simulink model "Hinf_sym"  (R2023a)
settings: Solver=VariableStepAuto  StartTime=0.0  StopTime=100  RelTol=1e-3
InitFcn:
  | %Hinf_init
values from neighbouring files (symbols this model uses):
  C = [1 0 0 0; 0 1 0 0]    [Hinf_1DOF.m]    (also in Hinf_2DOFinit.m; Hinf_U_init.m; Hinf_WU_init.m; Hinf_init.m)
  dtheta_0 = 0    [Hinf_1DOF.m]    (also in Hinf_2DOFinit.m; Hinf_U_init.m; Hinf_WU_init.m; Hinf_init.m)
  dz_0 = 0    [Hinf_1DOF.m]    (also in Hinf_2DOFinit.m; Hinf_U_init.m; Hinf_WU_init.m; Hinf_init.m)
  fa_w = 0    [Hinf_1DOF.m]    (also in Hinf_2DOFinit.m; Hinf_U_init.m; Hinf_WU_init.m; Hinf_init.m)
  fm_w = s_param.g*s_param.m    [Hinf_1DOF.m]    (also in Hinf_2DOFinit.m; Hinf_U_init.m; Hinf_WU_init.m; Hinf_init.m)
  K = tf(ss(K.A,K.B,K.C,K.D))    [Hinf_U_init.m]    (also in Hinf_WU_init.m; Hinf_init.m = tf(K))
  Km1 = 1.1    [Hinf_1DOF.m]    (also in Hinf_2DOFinit.m; Hinf_U_init.m; Hinf_WU_init.m; Hinf_init.m)
  Km1_real = Km1 + std_dev_Km*randn(1,1)    [Hinf_1DOF.m]    (also in Hinf_2DOFinit.m; Hinf_U_init.m; Hinf_WU_init.m; Hinf_init.m)
  Km2 = 1.1    [Hinf_1DOF.m]    (also in Hinf_2DOFinit.m; Hinf_U_init.m; Hinf_WU_init.m; Hinf_init.m)
  Km2_real = Km2 + std_dev_Km*randn(1,1)    [Hinf_1DOF.m]    (also in Hinf_2DOFinit.m; Hinf_U_init.m; Hinf_WU_init.m; Hinf_init.m)
  omega_d1 = 1    [Hinf_init.m]
  omega_d2 = 1    [Hinf_init.m]
  omega_y1 = 1e3    (= 1000)    [Hinf_WU_init.m]    (also in Hinf_init.m)
  omega_y2 = 1e3    (= 1000)    [Hinf_WU_init.m]    (also in Hinf_init.m)
  T1 = 0.05    [Hinf_1DOF.m]    (also in Hinf_2DOFinit.m; Hinf_U_init.m; Hinf_WU_init.m; Hinf_init.m)
  T1_real = T1 + std_dev_T*randn(1,1)    [Hinf_1DOF.m]    (also in Hinf_2DOFinit.m; Hinf_U_init.m; Hinf_WU_init.m; Hinf_init.m)
  T2 = 0.15    [Hinf_1DOF.m]    (also in Hinf_2DOFinit.m; Hinf_U_init.m; Hinf_WU_init.m; Hinf_init.m)
  T2_real = T2 + std_dev_T*randn(1,1)    [Hinf_1DOF.m]    (also in Hinf_2DOFinit.m; Hinf_U_init.m; Hinf_WU_init.m; Hinf_init.m)
  theta_0_real = theta_0 + std_dev.theta_0*randn(1,1)    [Hinf_1DOF.m]    (also in Hinf_2DOFinit.m = theta_0+std_dev.theta_0*randn(1,1); Hinf_U_init.m = theta_0+std_dev.theta_0*randn(1,1); Hinf_WU_init.m = theta_0+std_dev.theta_0*randn(1,1); Hinf_init.m = theta_0+std_dev.theta_0*randn(1,1))
  theta_w = 0    [Hinf_1DOF.m]    (also in Hinf_2DOFinit.m; Hinf_U_init.m; Hinf_WU_init.m; Hinf_init.m)
  Tm1 = 1    [Hinf_1DOF.m]    (also in Hinf_2DOFinit.m; Hinf_U_init.m; Hinf_WU_init.m; Hinf_init.m)
  Tm1_real = Tm1 + std_dev_Tm*randn(1,1)    [Hinf_1DOF.m]    (also in Hinf_2DOFinit.m; Hinf_U_init.m; Hinf_WU_init.m; Hinf_init.m)
  Tm2 = 1    [Hinf_1DOF.m]    (also in Hinf_2DOFinit.m; Hinf_U_init.m; Hinf_WU_init.m; Hinf_init.m)
  Tm2_real = Tm2 + std_dev_Tm*randn(1,1)    [Hinf_1DOF.m]    (also in Hinf_2DOFinit.m; Hinf_U_init.m; Hinf_WU_init.m; Hinf_init.m)
  z_0_real = z_0 + std_dev.z_0*randn(1,1)    [Hinf_1DOF.m]    (also in Hinf_2DOFinit.m = z_0+std_dev.z_0*randn(1,1); Hinf_U_init.m = z_0+std_dev.z_0*randn(1,1); Hinf_WU_init.m = z_0+std_dev.z_0*randn(1,1); Hinf_init.m = z_0+std_dev.z_0*randn(1,1))
  z_w = 200    [Hinf_1DOF.m]    (also in Hinf_2DOFinit.m = 400; Hinf_U_init.m = 400; Hinf_WU_init.m = 400; Hinf_init.m = 400)
undefined symbols (not defined in the file or in its folder): s_param, s_param_r, std_dev
libraries: simulink x4
settings Model: Creator=franc  LastModifiedBy=franc

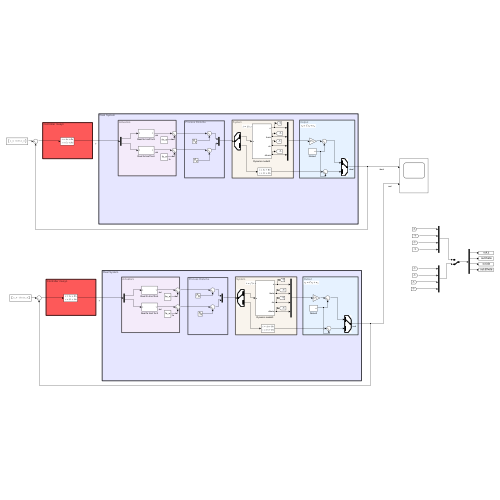
[thumbnail: Simulink's stored preview of the top-level diagram]
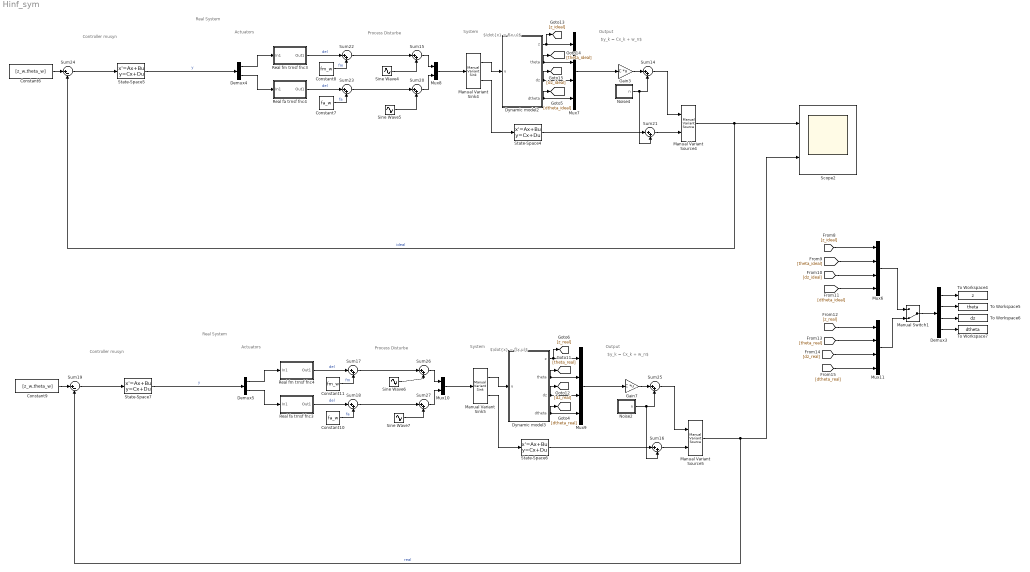
== system Hinf_sym ==
  note: $\dot{x} = f(x,u)$
  note: Controller musyn
  note: Real System
  note: Actuators
  note: Output
  note: Process Disturbe
  note: Controller musyn
  note: $y_k = Cx_k + w_n$
  note: System
  note: Process Disturbe
  note: $\dot{x} = f(x,u)$
  note: Actuators
  note: $y_k = Cx_k + w_n$
  note: Output
  note: System
  note: Real System
  Constant10 : Constant  Value=fa_w
  Constant11 : Constant  Value=fm_w
  Constant6 : Constant  Value=[z_w,theta_w]
  Constant7 : Constant  Value=fa_w
  Constant8 : Constant  Value=fm_w
  Constant9 : Constant  Value=[z_w,theta_w]
  Demux3 : Demux
  Demux4 : Demux  Outputs=2
  Demux5 : Demux  Outputs=2
  Dynamic model2 : Subsystem
  Dynamic model3 : Subsystem
  Gain3 : Gain  Gain=C  Multiplication=Matrix(K*u)
  Gain7 : Gain  Gain=C  Multiplication=Matrix(K*u)
  Manual Variant Sink4 : simulink/Signal Routing/Manual Variant Sink  NumChoices=2  LabelModeActiveChoice=V_1
  Manual Variant Sink5 : simulink/Signal Routing/Manual Variant Sink  NumChoices=2  LabelModeActiveChoice=V_1
  Manual Variant Source4 : simulink/Signal Routing/Manual Variant Source  NumChoices=2  LabelModeActiveChoice=V_1
  Manual Variant Source5 : simulink/Signal Routing/Manual Variant Source  NumChoices=2  LabelModeActiveChoice=V_1
  Manual Switch1 : ManualSwitch  CurrentSetting=0
  Mux10 : Mux  Inputs=2
  Mux{6..7,9,11} (4 alike) : Mux
  Mux8 : Mux  Inputs=2
  Noise2 : Subsystem
  Noise4 : Subsystem
  Real fa trnsf fnc3 : Subsystem
  Real fa trnsf fnc4 : Subsystem
  Real fm trnsf fnc3 : Subsystem
  Real fm trnsf fnc4 : Subsystem
  Scope2 : Scope  NumInputPorts=2
  Sine Wave4 : Sin  Amplitude=randn(1,1)*std_dev.fm  Frequency=omega_d1  SampleTime=0
  Sine Wave5 : Sin  Amplitude=randn(1,1)*std_dev.fa  Frequency=omega_d2  SampleTime=0
  Sine Wave6 : Sin  Amplitude=randn(1,1)*std_dev.fm  Frequency=omega_d1  SampleTime=0
  Sine Wave7 : Sin  Amplitude=randn(1,1)*std_dev.fa  Frequency=omega_d2  SampleTime=0
  State-Space4 : StateSpace  InitialCondition=0
  State-Space5 : StateSpace  A=K.A  B=K.B  C=K.C  D=K.D  InitialCondition=0
  State-Space6 : StateSpace  InitialCondition=0
  State-Space7 : StateSpace  A=K.A  B=K.B  C=K.C  D=K.D  InitialCondition=0
  Sum{14..18,20..23,25..27} (12 alike) : Sum  Inputs=|++
  Sum19 : Sum  Inputs=|+-
  Sum24 : Sum  Inputs=|+-
  To Workspace4 : ToWorkspace  VariableName=z  SaveFormat=Timeseries  SampleTime=-1
  To Workspace5 : ToWorkspace  VariableName=theta  SaveFormat=Timeseries  SampleTime=-1
  To Workspace6 : ToWorkspace  VariableName=dz  SaveFormat=Timeseries  SampleTime=-1
  To Workspace7 : ToWorkspace  VariableName=dtheta  SaveFormat=Timeseries  SampleTime=-1
  wires:
  Dynamic model2/1(z) -> [z_ideal], Mux7/1
  [theta_real] -> Mux11/2
  [dtheta_ideal] -> Mux6/4
  Mux6/1 -> Manual Switch1/1
  Sum21/1 -> Manual Variant Source4/2
  [z_ideal] -> Mux6/1
  Dynamic model3/1(z) -> Mux9/1, [z_real]
  Sum15/1 -> Mux8/1
  [z_real] -> Mux11/1
  [dtheta_real] -> Mux11/4
  Sum26/1 -> Mux10/1
  Demux3/1 -> To Workspace4/1
  Constant7/1 -> Sum23/2  "fa"
  Manual Variant Sink4/2 -> State-Space4/1
  Sum25/1 -> Manual Variant Source5/1
  Demux5/2 -> Real fa trnsf fnc3/1(In1)
  Real fa trnsf fnc3/1(Out1) -> Sum18/1  "del"
  Manual Variant Sink5/1 -> Dynamic model3/1(u)
  [dz_real] -> Mux11/3
  Demux3/2 -> To Workspace5/1
  Demux3/4 -> To Workspace7/1
  Sum16/1 -> Manual Variant Source5/2
  Mux11/1 -> Manual Switch1/2
  [theta_ideal] -> Mux6/2
  Manual Switch1/1 -> Demux3/1
  Demux3/3 -> To Workspace6/1
  Gain3/1 -> Sum14/1
  Constant10/1 -> Sum18/2  "fa"
  Dynamic model2/4(dtheta) -> Mux7/4, [dtheta_ideal]
  Sum19/1 -> State-Space7/1
  Manual Variant Sink5/2 -> State-Space6/1
  Sum22/1 -> Sum15/1
  Constant9/1 -> Sum19/1
  Sine Wave7/1 -> Sum27/2
  Sum20/1 -> Mux8/2
  Noise2/1(n) -> Sum16/2, Sum25/2
  [dz_ideal] -> Mux6/3
  State-Space6/1 -> Sum16/1
  Manual Variant Source4/1 -> Sum24/2, Scope2/1  "ideal"
  Sum23/1 -> Sum20/1
  Sum27/1 -> Mux10/2
  Real fm trnsf fnc4/1(Out1) -> Sum17/1  "del"
  Sine Wave5/1 -> Sum20/2
  Demux5/1 -> Real fm trnsf fnc4/1(In1)
  Real fm trnsf fnc3/1(Out1) -> Sum22/1  "del"
  Sum24/1 -> State-Space5/1
  Gain7/1 -> Sum25/1
  Mux10/1 -> Manual Variant Sink5/1
  Dynamic model3/2(theta) -> [theta_real], Mux9/2
  Constant6/1 -> Sum24/1
  Dynamic model3/3(dz) -> [dz_real], Mux9/3
  State-Space7/1 -> Demux5/1  "y"
  State-Space5/1 -> Demux4/1  "y"
  Mux9/1 -> Gain7/1
  Demux4/1 -> Real fm trnsf fnc3/1(In1)
  Dynamic model3/4(dtheta) -> [dtheta_real], Mux9/4
  Noise4/1(n) -> Sum14/2, Sum21/2
  State-Space4/1 -> Sum21/1
  Sum14/1 -> Manual Variant Source4/1
  Dynamic model2/2(theta) -> Mux7/2, [theta_ideal]
  Dynamic model2/3(dz) -> Mux7/3, [dz_ideal]
  Sum17/1 -> Sum26/1
  Manual Variant Source5/1 -> Scope2/2, Sum19/2  "real"
  Mux8/1 -> Manual Variant Sink4/1
  Sum18/1 -> Sum27/1
  Constant8/1 -> Sum22/2  "fm"
  Demux4/2 -> Real fa trnsf fnc4/1(In1)
  Mux7/1 -> Gain3/1
  Manual Variant Sink4/1 -> Dynamic model2/1(u)
  Real fa trnsf fnc4/1(Out1) -> Sum23/1  "del"
  Constant11/1 -> Sum17/2  "fm"
  Sine Wave4/1 -> Sum15/2
  Sine Wave6/1 -> Sum26/2

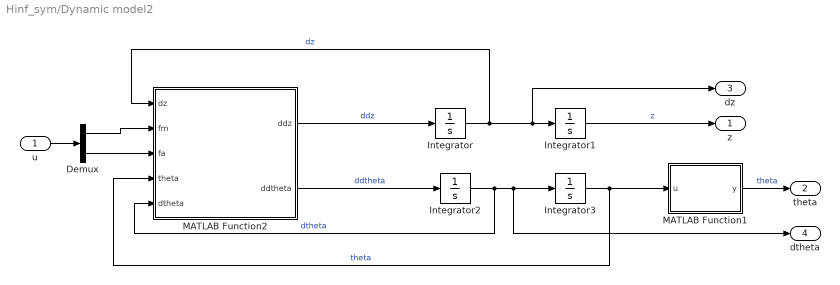
== system Hinf_sym/Dynamic model2 ==
  u : Inport
  Demux : Demux  Outputs=2
  Integrator : Integrator  InitialCondition=dz_0
  Integrator1 : Integrator  InitialCondition=z_0_real
  Integrator2 : Integrator  InitialCondition=dtheta_0
  Integrator3 : Integrator  InitialCondition=theta_0_real
  MATLAB Function1 : MATLAB Function  TreatAsAtomicUnit=on
  MATLAB Function2 : MATLAB Function  TreatAsAtomicUnit=on
  z : Outport
  theta : Outport  Port=2
  dz : Outport  Port=3
  dtheta : Outport  Port=4
  wires:
  Integrator3/1 -> MATLAB Function2/4(theta), MATLAB Function1/1(u)  "theta"
  Integrator2/1 -> dtheta/1, Integrator3/1, MATLAB Function2/5(dtheta)  "dtheta"
  MATLAB Function1/1(y) -> theta/1  "theta"
  Integrator1/1 -> z/1  "z"
  MATLAB Function2/2(ddtheta) -> Integrator2/1  "ddtheta"
  MATLAB Function2/1(ddz) -> Integrator/1  "ddz"
  Integrator/1 -> dz/1, Integrator1/1, MATLAB Function2/1(dz)  "dz"
  u/1 -> Demux/1
  Demux/2 -> MATLAB Function2/3(fa)
  Demux/1 -> MATLAB Function2/2(fm)

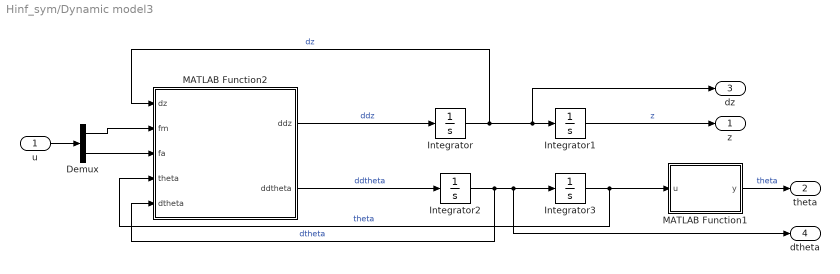
== system Hinf_sym/Dynamic model3 ==
  u : Inport
  Demux : Demux  Outputs=2
  Integrator : Integrator  InitialCondition=dz_0
  Integrator1 : Integrator  InitialCondition=z_0_real
  Integrator2 : Integrator  InitialCondition=dtheta_0
  Integrator3 : Integrator  InitialCondition=theta_0_real
  MATLAB Function1 : MATLAB Function  TreatAsAtomicUnit=on
  MATLAB Function2 : MATLAB Function  TreatAsAtomicUnit=on
  z : Outport
  theta : Outport  Port=2
  dz : Outport  Port=3
  dtheta : Outport  Port=4
  wires:
  Demux/1 -> MATLAB Function2/2(fm)
  Demux/2 -> MATLAB Function2/3(fa)
  u/1 -> Demux/1
  Integrator/1 -> MATLAB Function2/1(dz), Integrator1/1, dz/1  "dz"
  MATLAB Function2/1(ddz) -> Integrator/1  "ddz"
  MATLAB Function2/2(ddtheta) -> Integrator2/1  "ddtheta"
  Integrator1/1 -> z/1  "z"
  MATLAB Function1/1(y) -> theta/1  "theta"
  Integrator2/1 -> MATLAB Function2/5(dtheta), Integrator3/1, dtheta/1  "dtheta"
  Integrator3/1 -> MATLAB Function1/1(u), MATLAB Function2/4(theta)  "theta"

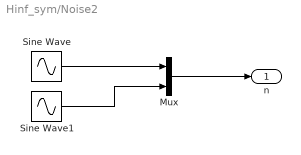
== system Hinf_sym/Noise2 ==
  Mux : Mux  Inputs=2
  Sine Wave : Sin  Amplitude=randn(1,1)*std_dev.y1  Frequency=omega_y1*10  SampleTime=0
  Sine Wave1 : Sin  Amplitude=randn(1,1)*std_dev.y2  Frequency=omega_y2*10  SampleTime=0
  n : Outport
  wires:
  Mux/1 -> n/1
  Sine Wave/1 -> Mux/1
  Sine Wave1/1 -> Mux/2

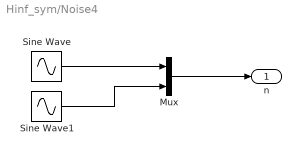
== system Hinf_sym/Noise4 ==
  Mux : Mux  Inputs=2
  Sine Wave : Sin  Amplitude=randn(1,1)*std_dev.y1  Frequency=omega_y1*10  SampleTime=0
  Sine Wave1 : Sin  Amplitude=randn(1,1)*std_dev.y2  Frequency=omega_y2*10  SampleTime=0
  n : Outport
  wires:
  Mux/1 -> n/1
  Sine Wave/1 -> Mux/1
  Sine Wave1/1 -> Mux/2

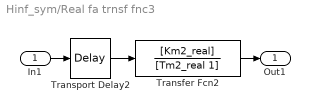
== system Hinf_sym/Real fa trnsf fnc3 ==
  In1 : Inport
  Transfer Fcn2 : TransferFcn  Numerator=[Km2_real]  Denominator=[Tm2_real 1]
  Transport Delay2 : TransportDelay  DelayTime=T2_real
  Out1 : Outport
  wires:
  In1/1 -> Transport Delay2/1
  Transfer Fcn2/1 -> Out1/1
  Transport Delay2/1 -> Transfer Fcn2/1

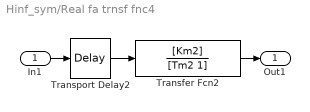
== system Hinf_sym/Real fa trnsf fnc4 ==
  In1 : Inport
  Transfer Fcn2 : TransferFcn  Numerator=[Km2]  Denominator=[Tm2 1]
  Transport Delay2 : TransportDelay  DelayTime=T2
  Out1 : Outport
  wires:
  Transport Delay2/1 -> Transfer Fcn2/1
  Transfer Fcn2/1 -> Out1/1
  In1/1 -> Transport Delay2/1

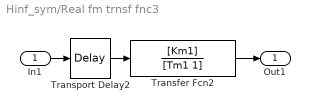
== system Hinf_sym/Real fm trnsf fnc3 ==
  In1 : Inport
  Transfer Fcn2 : TransferFcn  Numerator=[Km1]  Denominator=[Tm1 1]
  Transport Delay2 : TransportDelay  DelayTime=T1
  Out1 : Outport
  wires:
  In1/1 -> Transport Delay2/1
  Transfer Fcn2/1 -> Out1/1
  Transport Delay2/1 -> Transfer Fcn2/1

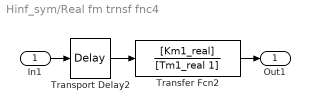
== system Hinf_sym/Real fm trnsf fnc4 ==
  In1 : Inport
  Transfer Fcn2 : TransferFcn  Numerator=[Km1_real]  Denominator=[Tm1_real 1]
  Transport Delay2 : TransportDelay  DelayTime=T1_real
  Out1 : Outport
  wires:
  Transport Delay2/1 -> Transfer Fcn2/1
  Transfer Fcn2/1 -> Out1/1
  In1/1 -> Transport Delay2/1

== matlab function Hinf_sym/Dynamic model2/MATLAB Function1 ==
  data: u input; y output
function y = fcn(u)

y = atan2(sin(u), cos(u));
end

== matlab function Hinf_sym/Dynamic model2/MATLAB Function2 ==
  data: dz input; fm input; fa input; ddz output; ddtheta output; theta input; dtheta input; s_param parameter
function [ddz, ddtheta] = fcn(dz, fm, fa, theta, dtheta, s_param)

% Rename params
J = s_param.J;     
m = s_param.m;     
b = s_param.b;      
beta = s_param.beta;    
g = s_param.g;     
l = s_param.l;   

%% Dynamic equations

ddz = -b/m * dz + fm/m * cos(theta) -g;
ddtheta = -beta/J * dtheta + 2 * l/J * fa;

end

== matlab function Hinf_sym/Dynamic model3/MATLAB Function1 ==
  data: u input; y output
function y = fcn(u)

y = atan2(sin(u), cos(u));
end

== matlab function Hinf_sym/Dynamic model3/MATLAB Function2 ==
  data: dz input; fm input; fa input; ddz output; ddtheta output; theta input; dtheta input; s_param parameter; s_param_r parameter
function [ddz, ddtheta] = fcn(dz, fm, fa, theta, dtheta, s_param, s_param_r)

% Rename params
J = s_param_r.J;     
m = s_param.m;     
b = s_param_r.b;      
beta = s_param_r.beta;    
g = s_param.g;     
l = s_param_r.l;   

%% Dynamic equations

ddz = -b/m * dz + fm/m * cos(theta) -g;
ddtheta = -beta/J * dtheta + 2 * l/J * fa;

end
